simulink model "CardioidBeamformer"  (R2019b)
settings: configuration reference "cset" (kept outside this file)
PostLoadFcn:
  | disp(['Executing PostLoadFcn in ' get_param(gcs,'Name')])
  | 
  | % Resize bus objects
  | hws = get_param(gcs, 'modelworkspace');
  | [SonarWorkbenchElementObj,SonarWorkbenchArrayObj,SonarWorkbenchBeamObj] = SetAcousticSensorDesignDimensions(hws.getVariable('Ne'),hws.getVariable('Ntype'),SonarWorkbenchElementObj,SonarWorkbenchArrayObj,SonarWorkbenchBeamObj);
model workspace (MAT data in the model file):
  Ne = 4
  Ntype = 2
values from neighbouring files (symbols this model uses):
  D = 4*pi/trapz(theta*pi/180,trapz(psi*pi/180,F,2))    [CalculateDI.m]    (also in CalculateJs.m = 2*pi/trapz(psi*pi/180,F); CalculateJv.m)
libraries: simulink_extras x2
settings Model: Creator=tom  LastModifiedBy=tom
settings ConfigSetRef: SourceName=cset  SourceLocation=Base Workspace

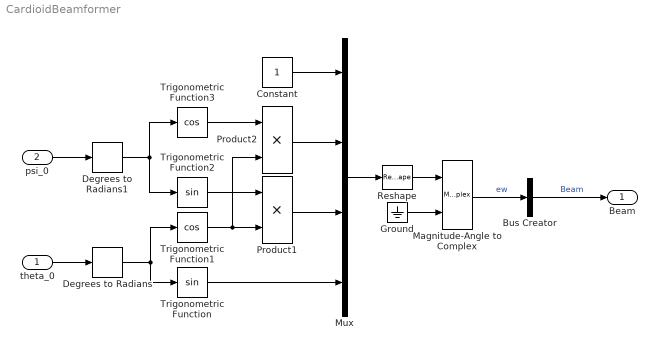
== system CardioidBeamformer ==
  theta_0 : Inport  OutDataTypeStr=double  Unit=deg  PortDimensions=1
  psi_0 : Inport  Port=2  OutDataTypeStr=double  Unit=deg  PortDimensions=1
  Bus Creator : BusCreator  Inputs=1  OutDataTypeStr=Bus: SonarWorkbenchBeamObj
  Constant : Constant  OutDataTypeStr=double
  Degrees to Radians : simulink_extras/Transformations/Degrees to Radians
  Degrees to Radians1 : simulink_extras/Transformations/Degrees to Radians
  Ground : Ground
  Magnitude-Angle to Complex : MagnitudeAngleToComplex
  Mux : Mux
  Product1 : Product
  Product2 : Product
  Reshape : Reshape  OutputDimensionality=Column vector (2-D)
  Trigonometric Function : Trigonometry
  Trigonometric Function1 : Trigonometry  Operator=cos
  Trigonometric Function2 : Trigonometry
  Trigonometric Function3 : Trigonometry  Operator=cos
  Beam : Outport  OutDataTypeStr=Bus: SonarWorkbenchBeamObj
  wires:
  Degrees to Radians1/1 -> Trigonometric Function3/1, Trigonometric Function2/1
  Constant/1 -> Mux/1
  psi_0/1 -> Degrees to Radians1/1
  Reshape/1 -> Magnitude-Angle to Complex/1
  Trigonometric Function1/1 -> Product2/2, Product1/2
  Mux/1 -> Reshape/1
  Degrees to Radians/1 -> Trigonometric Function1/1, Trigonometric Function/1
  Product2/1 -> Mux/2
  Trigonometric Function/1 -> Mux/4
  Magnitude-Angle to Complex/1 -> Bus Creator/1  "ew"
  Bus Creator/1 -> Beam/1  "Beam"
  theta_0/1 -> Degrees to Radians/1
  Trigonometric Function2/1 -> Product1/1
  Trigonometric Function3/1 -> Product2/1
  Ground/1 -> Magnitude-Angle to Complex/2
  Product1/1 -> Mux/3
